simulink model "mimo4"  (Simulink 3.00)
settings: Solver=ode45  SolverMode=SingleTasking  StartTime=0.0  StopTime=20  MaxStep=0.10  RelTol=1e-3  AbsTol=1e-3
settings Model: TimeSaveName=t  SaveOutput=off

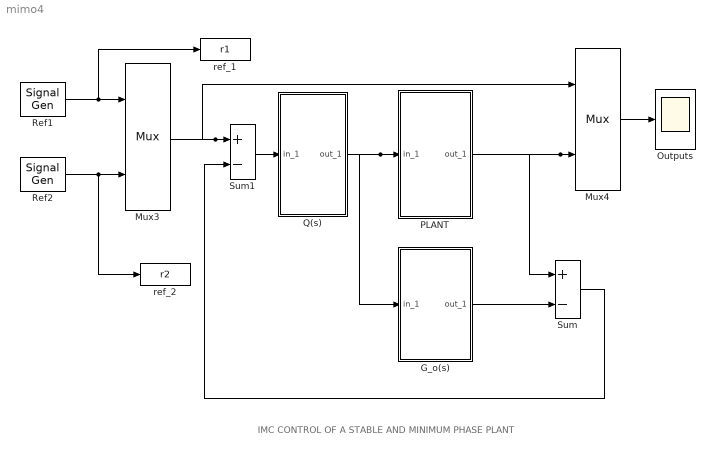
== system mimo4 ==
  note: IMC CONTROL OF A STABLE AND MINIMUM PHASE PLANT
  G_o(s) : Subsystem
      mask Type: Go(s)
      mask Display: disp('Go(s)')
  Mux3 : Mux  Inputs=2
      settings: DisplayOption=none
  Mux4 : Mux  Inputs=2
      settings: DisplayOption=none
  Outputs : Scope
      settings: TickLabels=on  TimeRange=20.000000  YMin=-2  YMax=2  SaveToWorkspace=off  SaveName=ScopeData  DataFormat=Matrix
  PLANT : Subsystem
      mask Type: Plant
      mask Display: disp('Plant')
  Q(s) : Subsystem
      mask Type: CONT
      mask Display: disp('CONT')
  Ref1 : SignalGenerator  WaveForm=square  Amplitude=1.000000  Frequency=1.000000  Units=rad/sec
  Ref2 : SignalGenerator  WaveForm=square  Amplitude=1.000000  Frequency=3.000000  Units=rad/sec
  Sum : Sum  Inputs=+-  SaturateOnIntegerOverflow=on
  Sum1 : Sum  Inputs=+-  SaturateOnIntegerOverflow=on
  ref_1 : ToWorkspace  VariableName=r1  SampleTime=0  SaveFormat=Matrix
      settings: Buffer=10000
  ref_2 : ToWorkspace  VariableName=r2  SampleTime=0  SaveFormat=Matrix
      settings: Buffer=10000
  wires:
  G_o(s)/1(out_1) -> Sum/2
  PLANT/1(out_1) -> Mux4/2, Sum/1
  Sum/1 -> Sum1/2
  Q(s)/1(out_1) -> PLANT/1(in_1), G_o(s)/1(in_1)
  Sum1/1 -> Q(s)/1(in_1)
  Ref1/1 -> Mux3/1, ref_1/1
  Ref2/1 -> Mux3/2, ref_2/1
  Mux3/1 -> Sum1/1, Mux4/1
  Mux4/1 -> Outputs/1

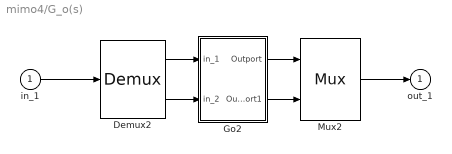
== system mimo4/G_o(s) ==
  in_1 : Inport  Port=1  PortWidth=-1  SampleTime=-1  DataType=auto
      settings: SignalType=auto
  Demux2 : Demux  Outputs=2
  Go2 : Subsystem
      mask Type: Go2
      mask Display: disp('Go2')
  Mux2 : Mux  Inputs=2
      settings: DisplayOption=none
  out_1 : Outport  Port=1  InitialOutput=0
  wires:
  Demux2/2 -> Go2/2(in_2)
  Demux2/1 -> Go2/1(in_1)
  Go2/2(Outport1) -> Mux2/2
  Go2/1(Outport) -> Mux2/1
  Mux2/1 -> out_1/1
  in_1/1 -> Demux2/1

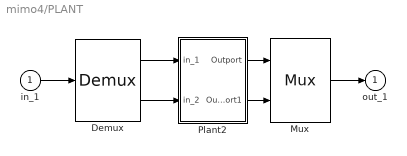
== system mimo4/PLANT ==
  in_1 : Inport  Port=1  PortWidth=-1  SampleTime=-1  DataType=auto
      settings: SignalType=auto
  Demux : Demux  Outputs=2
  Mux : Mux  Inputs=2
      settings: DisplayOption=none
  Plant2 : Subsystem
      mask Type: Plant2
      mask Display: disp('Plant2')
  out_1 : Outport  Port=1  InitialOutput=0
  wires:
  Demux/2 -> Plant2/2(in_2)
  Demux/1 -> Plant2/1(in_1)
  Plant2/2(Outport1) -> Mux/2
  Plant2/1(Outport) -> Mux/1
  Mux/1 -> out_1/1
  in_1/1 -> Demux/1

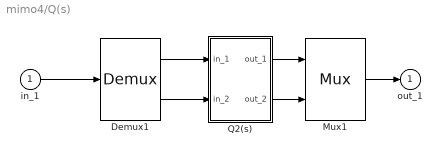
== system mimo4/Q(s) ==
  in_1 : Inport  Port=1  PortWidth=-1  SampleTime=-1  DataType=auto
      settings: SignalType=auto
  Demux1 : Demux  Outputs=2
  Mux1 : Mux  Inputs=2
      settings: DisplayOption=none
  Q2(s) : Subsystem
      mask Type: Q2(s)
      mask Display: disp('Q2(s)')
  out_1 : Outport  Port=1  InitialOutput=0
  wires:
  Demux1/2 -> Q2(s)/2(in_2)
  Demux1/1 -> Q2(s)/1(in_1)
  Q2(s)/2(out_2) -> Mux1/2
  Q2(s)/1(out_1) -> Mux1/1
  in_1/1 -> Demux1/1
  Mux1/1 -> out_1/1

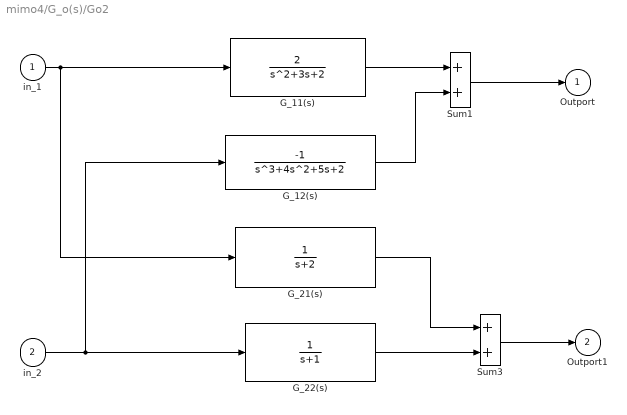
== system mimo4/G_o(s)/Go2 ==
  in_1 : Inport  Port=1  PortWidth=-1  SampleTime=-1  DataType=auto
      settings: SignalType=auto
  in_2 : Inport  Port=2  PortWidth=-1  SampleTime=-1  DataType=auto
      settings: SignalType=auto
  G_11(s) : TransferFcn  Numerator=2  Denominator=[1 3 2]
  G_12(s) : TransferFcn  Numerator=[-1]  Denominator="[1  4 5 2]"
  G_21(s) : TransferFcn  Numerator=1  Denominator=[1 2]
  G_22(s) : TransferFcn  Numerator=1  Denominator=[1 1]
  Sum1 : Sum  Inputs=++  SaturateOnIntegerOverflow=on
  Sum3 : Sum  Inputs=++  SaturateOnIntegerOverflow=on
  Outport : Outport  Port=1  InitialOutput=0
  Outport1 : Outport  Port=2  InitialOutput=0
  wires:
  Sum1/1 -> Outport/1
  G_11(s)/1 -> Sum1/1
  in_1/1 -> G_11(s)/1, G_21(s)/1
  G_12(s)/1 -> Sum1/2
  in_2/1 -> G_22(s)/1, G_12(s)/1
  G_22(s)/1 -> Sum3/2
  Sum3/1 -> Outport1/1
  G_21(s)/1 -> Sum3/1

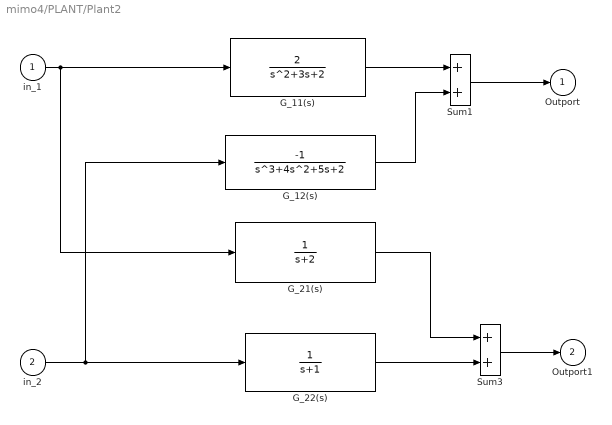
== system mimo4/PLANT/Plant2 ==
  in_1 : Inport  Port=1  PortWidth=-1  SampleTime=-1  DataType=auto
      settings: SignalType=auto
  in_2 : Inport  Port=2  PortWidth=-1  SampleTime=-1  DataType=auto
      settings: SignalType=auto
  G_11(s) : TransferFcn  Numerator=2  Denominator=[1 3 2]
  G_12(s) : TransferFcn  Numerator=[-1]  Denominator="[1  4 5 2]"
  G_21(s) : TransferFcn  Numerator=1  Denominator=[1 2]
  G_22(s) : TransferFcn  Numerator=1  Denominator=[1 1]
  Sum1 : Sum  Inputs=++  SaturateOnIntegerOverflow=on
  Sum3 : Sum  Inputs=++  SaturateOnIntegerOverflow=on
  Outport : Outport  Port=1  InitialOutput=0
  Outport1 : Outport  Port=2  InitialOutput=0
  wires:
  in_2/1 -> G_22(s)/1, G_12(s)/1
  G_22(s)/1 -> Sum3/2
  G_21(s)/1 -> Sum3/1
  Sum3/1 -> Outport1/1
  G_11(s)/1 -> Sum1/1
  in_1/1 -> G_11(s)/1, G_21(s)/1
  G_12(s)/1 -> Sum1/2
  Sum1/1 -> Outport/1

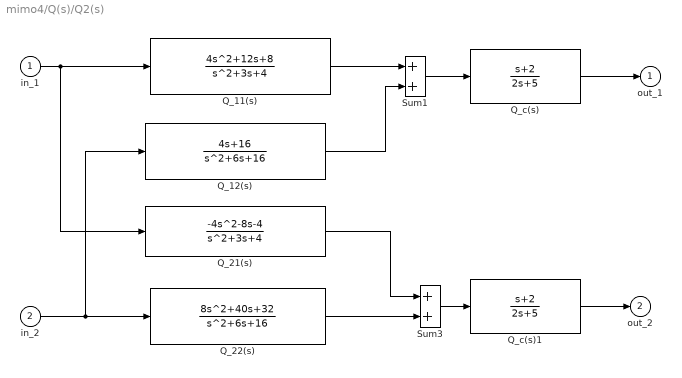
== system mimo4/Q(s)/Q2(s) ==
  in_1 : Inport  Port=1  PortWidth=-1  SampleTime=-1  DataType=auto
      settings: SignalType=auto
  in_2 : Inport  Port=2  PortWidth=-1  SampleTime=-1  DataType=auto
      settings: SignalType=auto
  Q_11(s) : TransferFcn  Numerator="[4  12 8]"  Denominator=[1 3 4]
  Q_12(s) : TransferFcn  Numerator=[4 16]  Denominator=[1 6 16]
  Q_21(s) : TransferFcn  Numerator=[-4 -8 -4]  Denominator=[1 3 4]
  Q_22(s) : TransferFcn  Numerator=[8 40 32]  Denominator=[1 6 16]
  Q_c(s) : TransferFcn  Numerator=[1 2]  Denominator="[2  5]"
  Q_c(s)1 : TransferFcn  Numerator=[1 2]  Denominator="[2  5]"
  Sum1 : Sum  Inputs=++  SaturateOnIntegerOverflow=on
  Sum3 : Sum  Inputs=++  SaturateOnIntegerOverflow=on
  out_1 : Outport  Port=1  InitialOutput=0
  out_2 : Outport  Port=2  InitialOutput=0
  wires:
  Q_11(s)/1 -> Sum1/1
  Q_21(s)/1 -> Sum3/1
  Q_22(s)/1 -> Sum3/2
  Q_12(s)/1 -> Sum1/2
  in_2/1 -> Q_22(s)/1, Q_12(s)/1
  in_1/1 -> Q_11(s)/1, Q_21(s)/1
  Sum1/1 -> Q_c(s)/1
  Sum3/1 -> Q_c(s)1/1
  Q_c(s)/1 -> out_1/1
  Q_c(s)1/1 -> out_2/1
